simulink model "devWeatherSimpleModel"  (R2018b)
settings: Solver=ode45  StartTime=0.0  StopTime=365*24*3600  RelTol=1e-3  EnableMultiTasking=on
libraries: Weather_Simple_Model x1, carnot x1
settings Model: Creator=drhf  LastModifiedBy=drhf
settings DataIOCC: LimitDataPoints=on  SaveFormat=Array  SignalLoggingSaveFormat=ModelDataLogs
settings OptimizationCC: ExpressionDepthLimit=2147483647  LifeSpan=inf
settings DebuggingCC: UnderspecifiedInitializationDetection=Classic  MergeDetectMultiDrivingBlocksExec=none  SolverPrmCheckMsg=warning  StateNameClashWarn=warning  SFUnexpectedBacktrackingDiag=warning  SFNoUnconditionalDefaultTransitionDiag=warning  SFExecutionAtInitializationDiag=none
settings HardwareCC: ProdBitPerPointer=32  ProdBitPerSizeT=32  ProdBitPerPtrDiffT=32  ProdLargestAtomicFloat=None  ProdIntDivRoundTo=Undefined  ProdEndianess=Unspecified  ProdWordSize=32  ProdHWDeviceType=32-bit Generic
settings ModelReferenceCC: PropagateSignalLabelsOutOfModel=off
settings SFSimCC: SimUseLocalCustomCode=off
settings RTWCC: RTWUseLocalCustomCode=off
settings CodeAppCC: StateflowObjectComments=on
settings GRTTargetCC: TargetLangStandard=C89/C90 (ANSI)  GeneratePreprocessorConditionals=Disable all  CombineOutputUpdateFcns=off  GRTInterface=on
settings ConfigComp: CovMetricSettings=dw  CovHtmlReporting=on  CovSaveCumulativeToWorkspaceVar=on  CovSaveSingleToWorkspaceVar=on  CovExternalEMLEnable=off

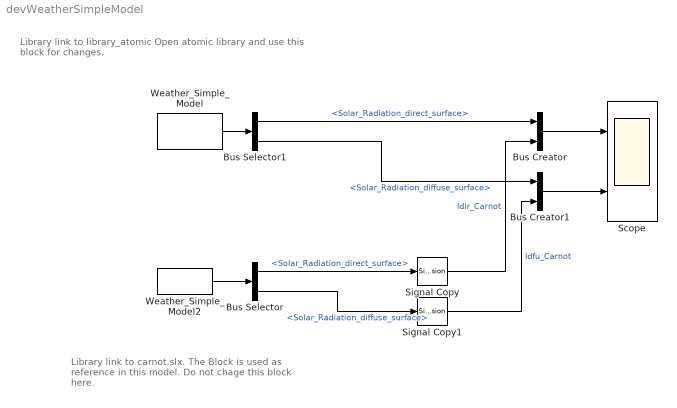
== system devWeatherSimpleModel ==
  note: Library link to carnot.slx. The Block
      | is used as reference in this model. Do
      | not chage this block here.
  note: Library link to library_atomic
      | Open atomic library and use this block for changes.
  Bus Creator : BusCreator  Inputs=2
  Bus Creator1 : BusCreator  Inputs=2
  Bus Selector : BusSelector  OutputSignals=Solar_Radiation_direct_surface,Solar_Radiation_diffuse_surface
  Bus Selector1 : BusSelector  OutputSignals=Solar_Radiation_direct_surface,Solar_Radiation_diffuse_surface
  Scope : Scope  NumInputPorts=2
  Signal Copy : SignalConversion  OverrideOpt=off
  Signal Copy1 : SignalConversion  OverrideOpt=off
  Weather_Simple_Model : Weather_Simple_Model/Weather_Simple_Model  Ibn=900  Idg=100  tamb=5  deltaTsky=-6  rh=50  precip="10e-3/24/3600           % 10 mm in 24 h"  cloud=0.125  p=1013e2  vw=1  wdir=270  lat=50  longi=0  timezone=0  colangle=0  colazi=0  colrot=0
  Weather_Simple_Model2 : carnot/Weather/Weather_Simple_Model  Ibn=900  Idg=100  tamb=5  deltaTsky=-6  rh=50  precip="10e-3/24/3600           % 10 mm in 24 h"  cloud=0.125  p=1013e2  vw=1  wdir=270  lat=50  colangle=0  colazi=0  colrot=0
      settings: SourceProductName=Carnot
  wires:
  Weather_Simple_Model2/1 -> Bus Selector/1
  Weather_Simple_Model/1 -> Bus Selector1/1
  Bus Selector1/1 -> Bus Creator/1  "<Solar_Radiation_direct_surface>"
  Bus Creator/1 -> Scope/1
  Bus Selector/1 -> Signal Copy/1  "<Solar_Radiation_direct_surface>"
  Signal Copy/1 -> Bus Creator/2  "Idir_Carnot"
  Bus Selector/2 -> Signal Copy1/1  "<Solar_Radiation_diffuse_surface>"
  Signal Copy1/1 -> Bus Creator1/2  "Idfu_Carnot"
  Bus Creator1/1 -> Scope/2
  Bus Selector1/2 -> Bus Creator1/1  "<Solar_Radiation_diffuse_surface>"
